simulink model "VictimTimingBlock"  (R2021b)
settings: Solver=VariableStepAuto  StartTime=0.0  StopTime=100e-3  RelTol=1e-3
values from neighbouring files (symbols this model uses):
  simulator = Simulator_revB()    [compute_sensed_targets.m]    (also in compute_sensed_values.m)
libraries: hdlsllib x4, simulink x2, phasedwavlib x1, dspswit3 x1
settings Model: Creator=David  LastModifiedBy=David

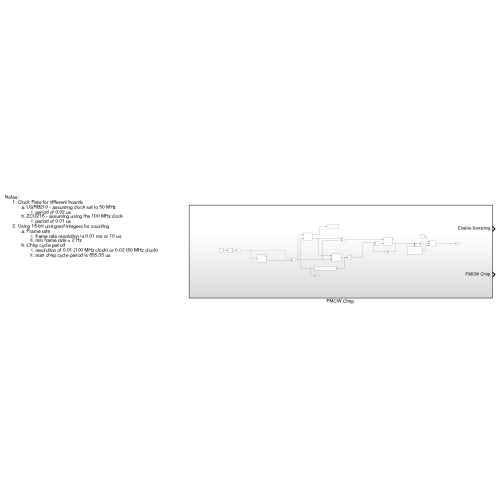
[thumbnail: Simulink's stored preview of the top-level diagram]
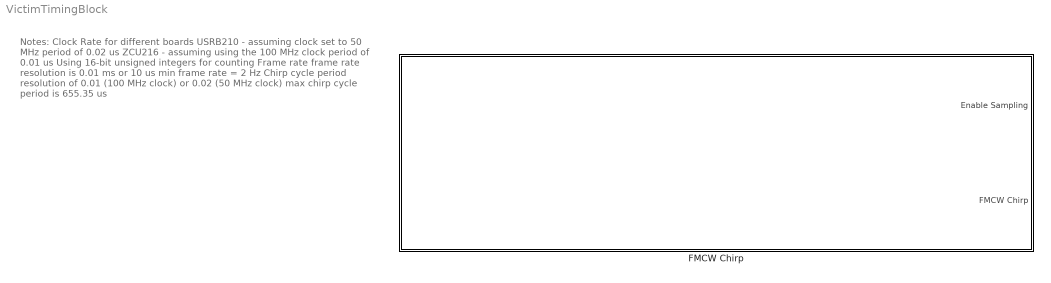
== system VictimTimingBlock ==
  note: Notes:
      | Clock Rate for different boards
      | USRB210 - assuming clock set to 50 MHz
      | period of 0.02 us
      | ZCU216 - assuming using the 100 MHz clock
      | period of 0.01 us
      | Using 16-bit unsigned integers for counting
      | Frame rate
      | frame rate resolution is 0.01 ms or 10 us
      | min frame rate = 2 Hz
      | Chirp cycle period
      | resolution of 0.01 (100 MHz clock) or 0.02 (50 MHz clock)
      | max chirp cycle period is 655.35 us
  FMCW Chirp : Subsystem

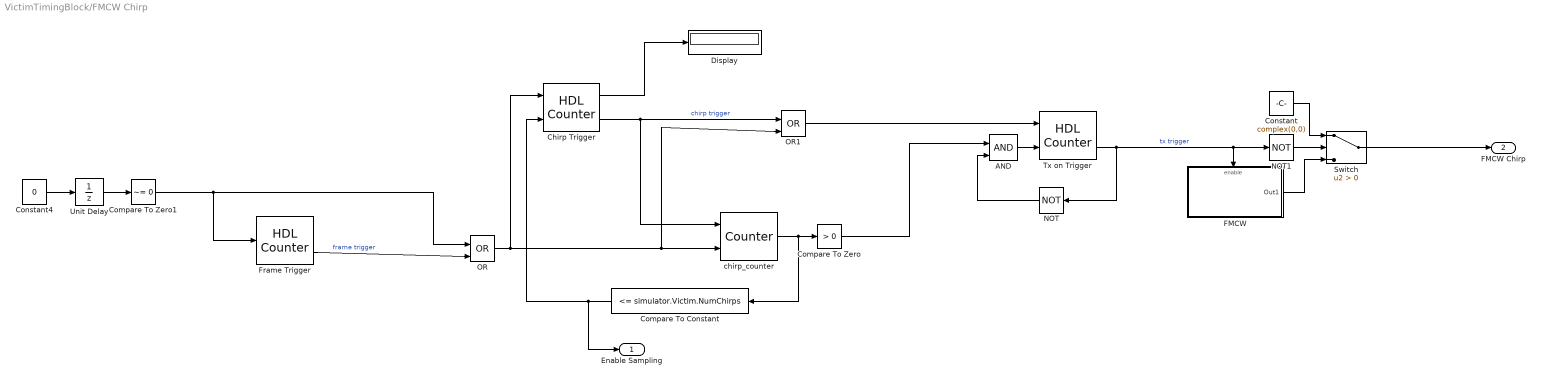
== system VictimTimingBlock/FMCW Chirp ==
  AND : Logic  IconShape=distinctive  AllPortsSameDT=off  OutDataTypeStr=boolean
  Chirp Trigger : hdlsllib/Sources/HDL Counter  CountType=Count limited  CountInit=1  CountStep=1  CountMax=simulator.Victim.FMCW_sampling_rate_Hz * simulator.Victim.sweep_time + simulator.Victim.num_samples_idle_time  CountFromType=Initial value  CountFrom=1  CountResetPort=on  CountLoadPort=off  CountEnbPort=on  CountDirPort=off  CountHitOutputPort=on  CountDataType=Unsigned  CountWordLen=16  CountFracLen=0  CountSampTime=1
  Compare To Constant : simulink/Logic and Bit Operations/Compare To Constant  relop=<=  const=simulator.Victim.NumChirps  OutDataTypeStr=boolean
  Compare To Zero : hdlsllib/Logic and Bit Operations/Compare To Zero  relop=>  OutDataTypeStr=boolean
      settings: SourceProductBaseCode=SL
  Compare To Zero1 : simulink/Logic and Bit Operations/Compare To Zero  relop=~=  OutDataTypeStr=boolean
  Constant : Constant  Value=complex(0,0)
  Constant4 : Constant  Value=0
  Display : Display
  FMCW : Subsystem
  Frame Trigger : hdlsllib/Sources/HDL Counter  CountType=Count limited  CountInit=1  CountStep=1  CountMax=simulator.Victim.num_samples_per_frame  CountFromType=Initial value  CountFrom=1  CountResetPort=on  CountLoadPort=off  CountEnbPort=off  CountDirPort=off  CountHitOutputPort=on  CountDataType=Unsigned  CountWordLen=32  CountFracLen=0  CountSampTime=1
  NOT : Logic  Operator=NOT  IconShape=distinctive  AllPortsSameDT=off  OutDataTypeStr=boolean
  NOT1 : Logic  Operator=NOT  IconShape=distinctive  AllPortsSameDT=off  OutDataTypeStr=boolean
  OR : Logic  Operator=OR  IconShape=distinctive  AllPortsSameDT=off  OutDataTypeStr=boolean
  OR1 : Logic  Operator=OR  IconShape=distinctive  AllPortsSameDT=off  OutDataTypeStr=boolean
  Switch : Switch  Criteria=u2 > Threshold
  Tx on Trigger : hdlsllib/Sources/HDL Counter  CountType=Count limited  CountInit=1  CountStep=1  CountMax=simulator.Victim.num_samples_idle_time  CountFromType=Initial value  CountFrom=1  CountResetPort=on  CountLoadPort=off  CountEnbPort=on  CountDirPort=off  CountHitOutputPort=on  CountDataType=Unsigned  CountWordLen=16  CountFracLen=0  CountSampTime=1
  Unit Delay : UnitDelay  InitialCondition=1  SampleTime=-1  HasFrameUpgradeWarning=on
  chirp_counter : dspswit3/Counter  Direction=Up  CountEvent=Rising edge  CounterSize=User defined  MaxCount=simulator.Victim.NumChirps + 1  InitialCount=1  Output=Count  HitValue=32  ResetInput=on  SamplesPerFrame=1  Ts=1  CntDtype=int16  HitDtype=Logical
  Enable Sampling : Outport
  FMCW Chirp : Outport  Port=2
  wires:
  Switch/1 -> FMCW Chirp/1
  chirp_counter/1 -> Compare To Constant/1, Compare To Zero/1
  Tx on Trigger/2 -> NOT/1, FMCW/Enable, NOT1/1  "tx trigger"
  AND/1 -> Tx on Trigger/2
  FMCW/1(Out1) -> Switch/3
  NOT1/1 -> Switch/2
  Constant/1 -> Switch/1
  Chirp Trigger/2 -> chirp_counter/1, OR1/1  "chirp trigger"
  Compare To Zero/1 -> AND/1
  NOT/1 -> AND/2
  Compare To Constant/1 -> Enable Sampling/1, Chirp Trigger/2
  Frame Trigger/2 -> OR/2  "frame trigger"
  Compare To Zero1/1 -> Frame Trigger/1, OR/1
  OR/1 -> Chirp Trigger/1, OR1/2, chirp_counter/2
  OR1/1 -> Tx on Trigger/1
  Unit Delay/1 -> Compare To Zero1/1
  Constant4/1 -> Unit Delay/1
  Chirp Trigger/1 -> Display/1

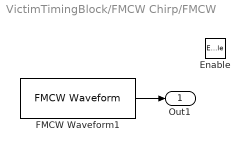
== system VictimTimingBlock/FMCW Chirp/FMCW ==
  Enable : EnablePort  StatesWhenEnabling=reset
  FMCW Waveform1 : phasedwavlib/FMCW Waveform  SampleRate=simulator.Victim.FMCW_sampling_rate_Hz  SweepTime=simulator.Victim.sweep_time  SweepBandwidth=simulator.Victim.Chirp_Tx_Bandwidth_MHz * 1e6  SweepDirection=Up  SweepInterval=Positive  OutputFormat=Samples  NumSamples=1  NumSweeps=waveform_params.num_sweeps  SimulateUsing=Interpreted execution
      settings: SourceProductBaseCode=AR
  Out1 : Outport
  wires:
  FMCW Waveform1/1 -> Out1/1
